simulink model "attitude_observer_test"  (R2016b)
settings: Solver=VariableStepAuto  StartTime=0.0  StopTime=10.0  RelTol=1e-3
settings Model: Creator=liana  LastModifiedBy=liana

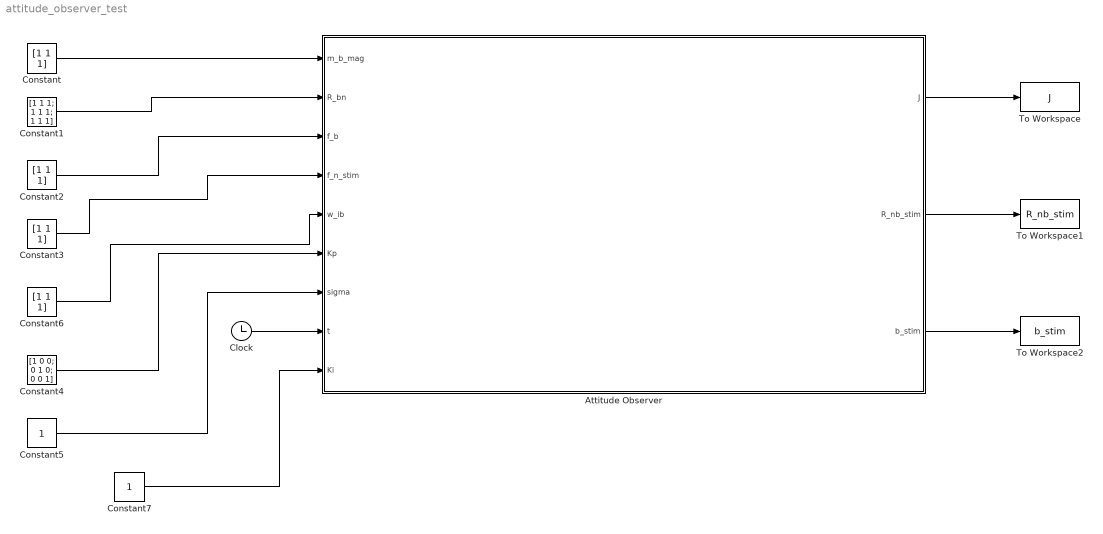
== system attitude_observer_test ==
  Attitude Observer : Subsystem
  Clock : Clock
  Constant{,2..3,6} (4 alike) : Constant  Value=[1 1 1]
  Constant1 : Constant  Value=[1 1 1; 1 1 1; 1 1 1]
  Constant4 : Constant  Value=[1 0 0; 0 1 0; 0 0 1]
  Constant5 : Constant
  Constant7 : Constant
  To Workspace : ToWorkspace  VariableName=J  SampleTime=-1
  To Workspace1 : ToWorkspace  VariableName=R_nb_stim  SampleTime=-1
  To Workspace2 : ToWorkspace  VariableName=b_stim  SampleTime=-1
  wires:
  Constant/1 -> Attitude Observer/1(m_b_mag)
  Constant1/1 -> Attitude Observer/2(R_bn)
  Constant2/1 -> Attitude Observer/3(f_b)
  Constant3/1 -> Attitude Observer/4(f_n_stim)
  Constant4/1 -> Attitude Observer/6(Kp)
  Constant5/1 -> Attitude Observer/7(sigma)
  Constant6/1 -> Attitude Observer/5(w_ib)
  Constant7/1 -> Attitude Observer/9(Ki)
  Clock/1 -> Attitude Observer/8(t)
  Attitude Observer/1(J) -> To Workspace/1
  Attitude Observer/2(R_nb_stim) -> To Workspace1/1
  Attitude Observer/3(b_stim) -> To Workspace2/1

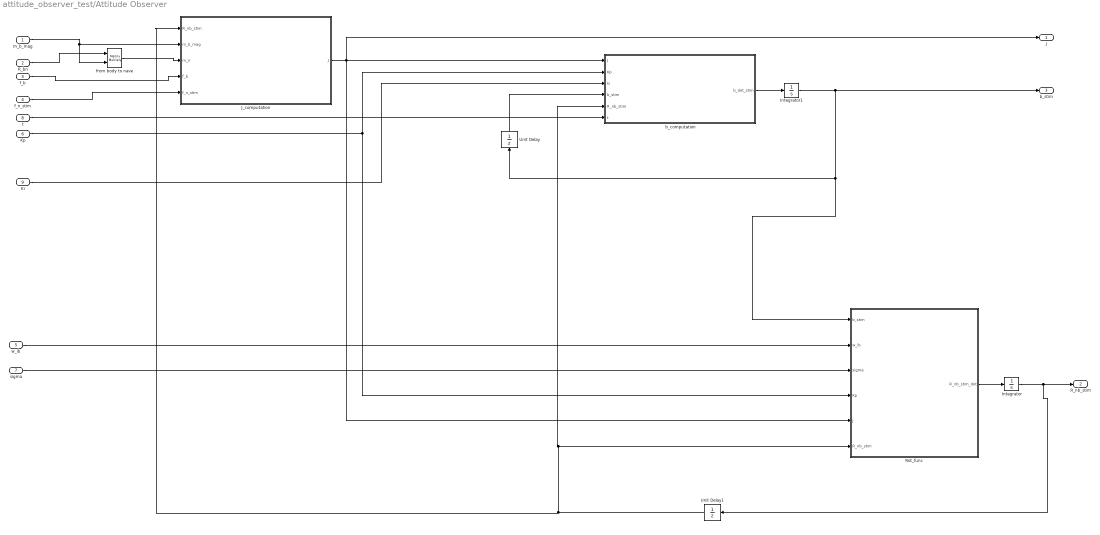
== system attitude_observer_test/Attitude Observer ==
  m_b_mag : Inport
  R_bn : Inport  Port=2
  f_b : Inport  Port=3
  f_n_stim : Inport  Port=4
  w_ib : Inport  Port=5
  Kp : Inport  Port=6
  sigma : Inport  Port=7
  t : Inport  Port=8
  Ki : Inport  Port=9
  Integrator : Integrator  InitialCondition=0.0000001
  Integrator1 : Integrator
  J_computation : Subsystem
  Rot_func : MATLAB Function  TreatAsAtomicUnit=on
  Unit Delay : UnitDelay  SampleTime=-1
  Unit Delay1 : UnitDelay  SampleTime=-1
  b_computation : MATLAB Function  TreatAsAtomicUnit=on
  from body to nave : Product  Multiplication=Matrix(*)
  J : Outport
  R_nb_stim : Outport  Port=2
  b_stim : Outport  Port=3
  wires:
  m_b_mag/1 -> from body to nave/2, J_computation/2(m_b_mag)
  Rot_func/1(R_nb_stim_dot) -> Integrator/1
  b_computation/1(b_dot_stim) -> Integrator1/1
  Integrator1/1 -> Unit Delay/1, Rot_func/1(b_stim), b_stim/1
  from body to nave/1 -> J_computation/3(m_n)
  f_b/1 -> J_computation/4(f_b)
  f_n_stim/1 -> J_computation/5(f_n_stim)
  J_computation/1(J) -> J/1, Rot_func/5(J), b_computation/1(J)
  Kp/1 -> Rot_func/4(Kp), b_computation/2(Kp)
  Ki/1 -> b_computation/3(ki)
  sigma/1 -> Rot_func/3(sigma)
  w_ib/1 -> Rot_func/2(w_ib)
  R_bn/1 -> from body to nave/1
  t/1 -> b_computation/6(t)
  Integrator/1 -> R_nb_stim/1, Unit Delay1/1
  Unit Delay/1 -> b_computation/4(b_stim)
  Unit Delay1/1 -> J_computation/1(R_nb_stim), b_computation/5(R_nb_stim), Rot_func/6(R_nb_stim)

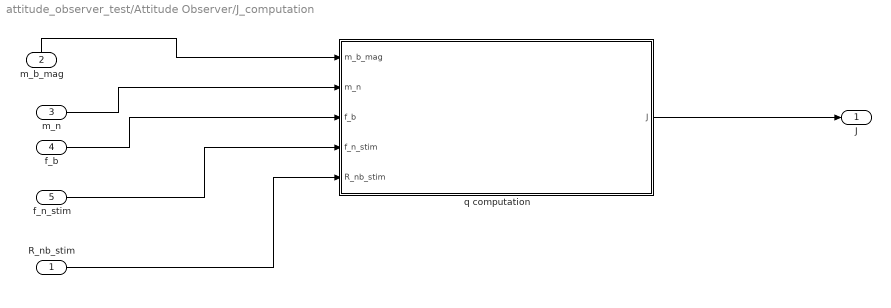
== system attitude_observer_test/Attitude Observer/J_computation ==
  R_nb_stim : Inport
  m_b_mag : Inport  Port=2
  m_n : Inport  Port=3
  f_b : Inport  Port=4
  f_n_stim : Inport  Port=5
  q computation : MATLAB Function  TreatAsAtomicUnit=on
  J : Outport
  wires:
  m_n/1 -> q computation/2(m_n)
  f_n_stim/1 -> q computation/4(f_n_stim)
  m_b_mag/1 -> q computation/1(m_b_mag)
  f_b/1 -> q computation/3(f_b)
  q computation/1(J) -> J/1
  R_nb_stim/1 -> q computation/5(R_nb_stim)

== matlab function attitude_observer_test/Attitude Observer/J_computation/q computation ==
  data: m_b_mag input; m_n input; f_b input; f_n_stim input size=3; J output; R_nb_stim input size=[3,3]
function J  = qEfunc(m_b_mag, m_n, f_b, f_n_stim, R_nb_stim)

g_n = [0 0 9.81]';

q1_b = m_b_mag/norm(m_b_mag,2);
q2_b = f_b/norm(g_n,2);

q1_n = m_n/norm(m_n,2);
q2_n = f_n_stim/norm(g_n,2);


E_b = [q1_b, skew(q1_b)*q2_b, (skew(q1_b)*skew(q1_b))*q2_b];
E_n = [q1_n, skew(q1_n)*q2_n, (skew(q1_n)*skew(q1_n))*q2_n];

J = (E_n - R_nb_stim * E_b) * (E_b');

end

== matlab function attitude_observer_test/Attitude Observer/b_computation ==
  data: J input; b_dot_stim output size=3; Kp input; ki input; b_stim input; R_nb_stim input; t input
function b_dot_stim = b_dot_stim_func(J, Kp, ki, b_stim, R_nb_stim, t)

% don't break balls if there are too rows

%b_dot_stim = zeros(3 ,1);

if t == 0
   
    b_stim = zeros(3, 1);
    
end

SAT = sat(R_nb_stim)';
PA = pa( SAT * Kp * J);
VEX = vexfunc(PA);
b_dot_stim = Proj(b_stim , (-ki * VEX));

end

== matlab function attitude_observer_test/Attitude Observer/Rot_func ==
  data: b_stim input; R_nb_stim_dot output; w_ib input; sigma input; Kp input; J input; R_nb_stim input
function R_nb_stim_dot = rot_func(b_stim,w_ib,sigma,Kp,J,R_nb_stim) 

Skew = skew(w_ib - b_stim);

R_nb_stim_dot = R_nb_stim * Skew + sigma * Kp * J;

end
